simulink model "regulator"  (R2016a)
settings: Solver=ode45  StartTime=0.0  StopTime=10.0  RelTol=1e-3
values from neighbouring files (symbols this model uses):
  kp = mrowki(i,1)    [PSO.m]    (also in PSO_testy.m)
  Td = mrowki(i,3)    [PSO.m]    (also in PSO_testy.m)
  Ti = mrowki(i,2)    [PSO.m]    (also in PSO_testy.m)
settings Model: Creator=Michal  LastModifiedBy=Michal
settings DataIOCC: LimitDataPoints=on  SaveFormat=Array
settings HardwareCC: ProdBitPerPointer=32  ProdLargestAtomicFloat=None  ProdIntDivRoundTo=Undefined  ProdEndianess=Unspecified  ProdWordSize=32  ProdHWDeviceType=32-bit Generic
settings ModelReferenceCC: PropagateSignalLabelsOutOfModel=off
settings ConfigComp: CovModelRefEnable=Off

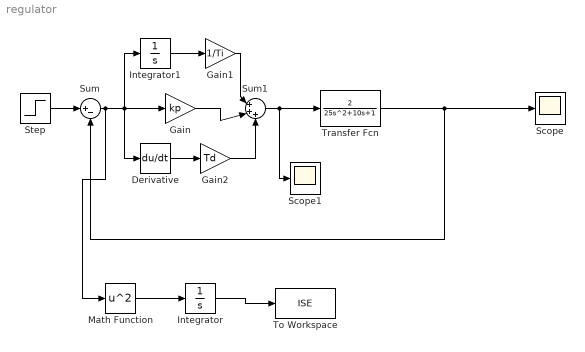
== system regulator ==
  Derivative : Derivative
  Gain : Gain  Gain=kp
  Gain1 : Gain  Gain=1/Ti
  Gain2 : Gain  Gain=Td
  Integrator : Integrator
  Integrator1 : Integrator
  Math Function : Math  Operator=square  SaturateOnIntegerOverflow=on
  Scope : Scope
  Scope1 : Scope
  Step : Step  SampleTime=0
  Sum : Sum  Inputs=|+-
  Sum1 : Sum  Inputs=|+++
  To Workspace : ToWorkspace  VariableName=ISE  SampleTime=-1
  Transfer Fcn : TransferFcn  Numerator=[2]  Denominator=[25 10 1]
  wires:
  Sum/1 -> Integrator1/1, Derivative/1, Gain/1, Math Function/1
  Transfer Fcn/1 -> Sum/2, Scope/1
  Step/1 -> Sum/1
  Math Function/1 -> Integrator/1
  Integrator/1 -> To Workspace/1
  Derivative/1 -> Gain2/1
  Integrator1/1 -> Gain1/1
  Gain1/1 -> Sum1/1
  Gain2/1 -> Sum1/3
  Gain/1 -> Sum1/2
  Sum1/1 -> Scope1/1, Transfer Fcn/1
